simulink model "Modelado_valvula"  (R2014a)
settings: Solver=ode45  StartTime=0.0  StopTime=60  RelTol=1e-3
values from neighbouring files (symbols this model uses):
  Ap0 = 49.978    [Seccion_5.m]
  Fh0 = 0.8946    [Seccion_5.m]
  k_v = 0.0179    [Seccion_5.m]
  tau_v = 3.5    [Seccion_5.m]
  tita_v = 0.9993    [Seccion_5.m]
settings Model: Creator=lraff  LastModifiedBy=lraff

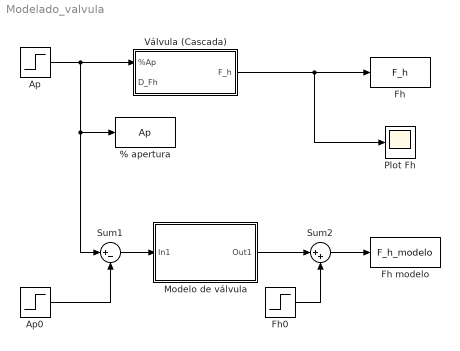
== system Modelado_valvula ==
  % apertura : ToWorkspace  VariableName=Ap  SaveFormat=Structure With Time
  Ap : Step  Time=10  Before=Ap0  After=Ap0*1.04  SampleTime=1
  Ap0 : Step  Time=0  Before=Ap0  After=Ap0  SampleTime=1
  Fh : ToWorkspace  VariableName=F_h  SaveFormat=Structure With Time
  Fh modelo : ToWorkspace  VariableName=F_h_modelo  SaveFormat=Structure With Time
  Fh0 : Step  Time=0  Before=Fh0  After=Fh0  SampleTime=1
  Modelo de válvula : Subsystem
  Plot Fh : Scope
  Sum1 : Sum  Inputs=|+-
  Sum2 : Sum  Inputs=|++
  Válvula (Cascada) : Subsystem
  wires:
  Válvula (Cascada)/1(F_h) -> Plot Fh/1, Fh/1
  Ap/1 -> Sum1/1, % apertura/1, Válvula (Cascada)/1(%Ap)
  Sum1/1 -> Modelo de válvula/1(In1)
  Ap0/1 -> Sum1/2
  Modelo de válvula/1(Out1) -> Sum2/1
  Sum2/1 -> Fh modelo/1
  Fh0/1 -> Sum2/2

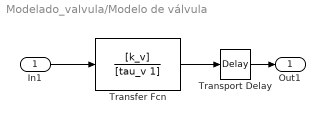
== system Modelado_valvula/Modelo de válvula ==
  In1 : Inport
  Transfer Fcn : TransferFcn  Numerator=[k_v]  Denominator=[tau_v 1]
  Transport Delay : TransportDelay  DelayTime=tita_v
  Out1 : Outport
  wires:
  Transfer Fcn/1 -> Transport Delay/1
  In1/1 -> Transfer Fcn/1
  Transport Delay/1 -> Out1/1

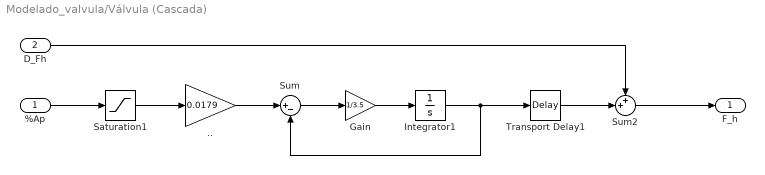
== system Modelado_valvula/Válvula (Cascada) ==
  %Ap : Inport
  D_Fh : Inport  Port=2
  .. : Gain  Gain=0.0179
  Gain : Gain  Gain=1/3.5
  Integrator1 : Integrator  InitialCondition=Fh0
  Saturation1 : Saturate  UpperLimit=100  LowerLimit=0
  Sum : Sum  Inputs=|+-
  Sum2 : Sum  Inputs=++|
  Transport Delay1 : TransportDelay  InitialOutput=Fh0
  F_h : Outport
  wires:
  D_Fh/1 -> Sum2/1
  Sum2/1 -> F_h/1
  %Ap/1 -> Saturation1/1
  Saturation1/1 -> ../1
  Sum/1 -> Gain/1
  Gain/1 -> Integrator1/1
  Integrator1/1 -> Transport Delay1/1, Sum/2
  ../1 -> Sum/1
  Transport Delay1/1 -> Sum2/2
